simulink model "simu"  (R2024b)
settings: Solver=VariableStepAuto  StartTime=0.0  StopTime=10.0  RelTol=1e-3
values from neighbouring files (symbols this model uses):
  den1 = [2 3]    [t1.m]
  den2 = [5 6]    [t1.m]
  num1 = [1]    [t1.m]
  num2 = [4]    [t1.m]
settings Model: Creator=Faizy  LastModifiedBy=Faizy

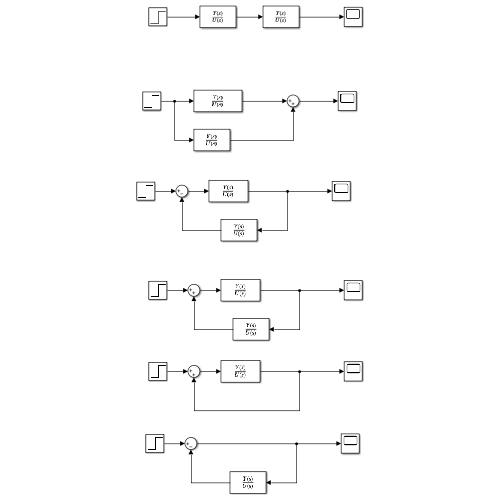
[thumbnail: Simulink's stored preview of the top-level diagram]
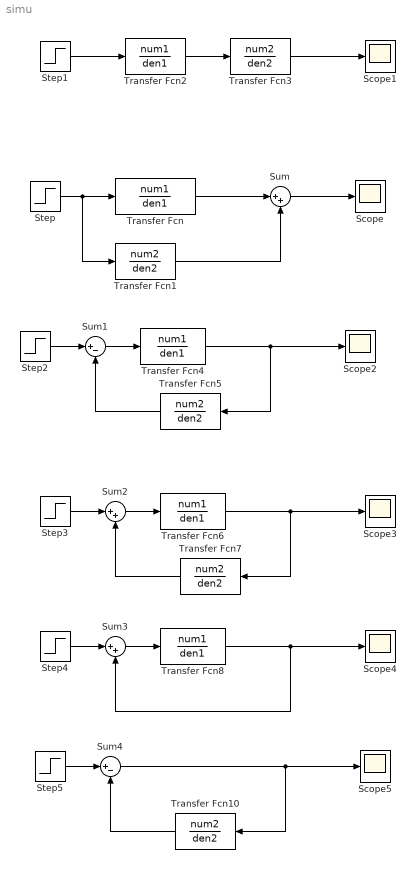
== system simu ==
  Scope{,1..5} (6 alike) : Scope
  Step{,1..5} (6 alike) : Step  SampleTime=0
  Sum : Sum  Inputs=|++
  Sum1 : Sum  Inputs=|+-
  Sum2 : Sum  Inputs=|++
  Sum3 : Sum  Inputs=|++
  Sum4 : Sum  Inputs=|+-
  Transfer Fcn{,2,4,6,8} (5 alike) : TransferFcn  Numerator=num1  Denominator=den1
  Transfer Fcn{1,3,5,7,10} (5 alike) : TransferFcn  Numerator=num2  Denominator=den2
  wires:
  Step/1 -> Transfer Fcn1/1, Transfer Fcn/1
  Transfer Fcn1/1 -> Sum/2
  Transfer Fcn/1 -> Sum/1
  Sum/1 -> Scope/1
  Step1/1 -> Transfer Fcn2/1
  Transfer Fcn2/1 -> Transfer Fcn3/1
  Transfer Fcn3/1 -> Scope1/1
  Sum1/1 -> Transfer Fcn4/1
  Step2/1 -> Sum1/1
  Transfer Fcn4/1 -> Transfer Fcn5/1, Scope2/1
  Transfer Fcn5/1 -> Sum1/2
  Sum2/1 -> Transfer Fcn6/1
  Transfer Fcn7/1 -> Sum2/2
  Transfer Fcn6/1 -> Transfer Fcn7/1, Scope3/1
  Step3/1 -> Sum2/1
  Transfer Fcn8/1 -> Sum3/2, Scope4/1
  Sum3/1 -> Transfer Fcn8/1
  Step4/1 -> Sum3/1
  Sum4/1 -> Transfer Fcn10/1, Scope5/1
  Step5/1 -> Sum4/1
  Transfer Fcn10/1 -> Sum4/2
